simulink model "tbm_ref"  (R2020a)
settings: configuration reference "config_10ms" (kept outside this file)
PreLoadFcn:
  | defParm_cu_tbm_spt
libraries: lib_decmp_Calib_tbm_brkBts_x8 x1, lib_decmp_Calib_tbm_ctr_x8 x1, lib_decmp_CtrSet_tbm_enab_x8 x1, lib_decmp_Calib_tbm_strDistb_x8 x1, lib_decmp_Calib_tbm_supCtr_x8 x1, lib_sig_fault_tolerate x1
settings Model: Creator=Administrator  LastModifiedBy=bowen.zheng
settings ConfigSetRef: SourceName=config_10ms  SourceLocation=Base Workspace

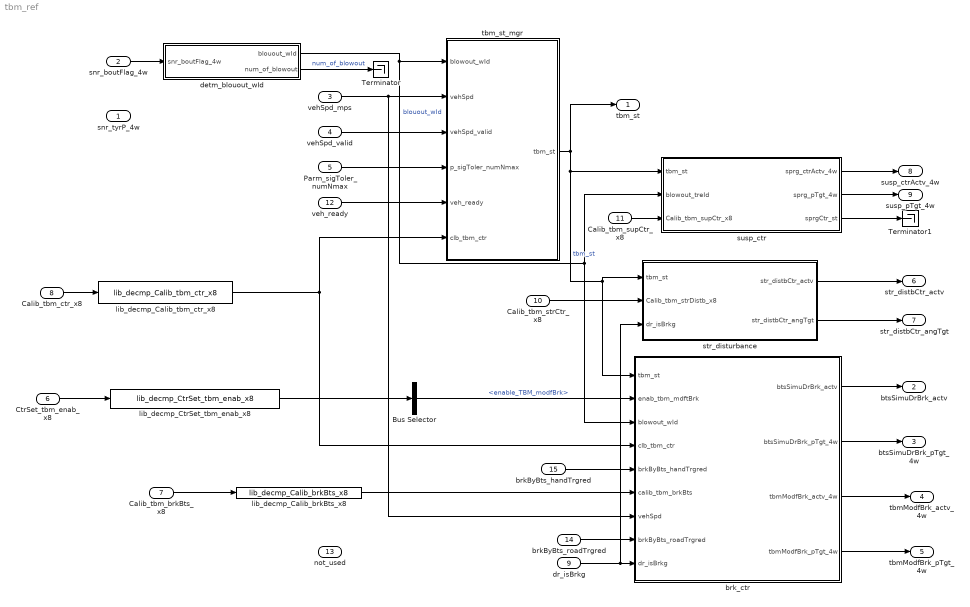
== system tbm_ref ==
  snr_tyrP_4w : Inport  OutDataTypeStr=single  PortDimensions=4
  snr_boutFlag_4w : Inport  Port=2  OutDataTypeStr=boolean  PortDimensions=4
  vehSpd_mps : Inport  Port=3  OutDataTypeStr=single  PortDimensions=1
  vehSpd_valid : Inport  Port=4  OutDataTypeStr=boolean  PortDimensions=1
  Parm_sigToler_numNmax : Inport  Port=5  OutDataTypeStr=int8  PortDimensions=2
  CtrSet_tbm_enab_x8 : Inport  Port=6  OutDataTypeStr=boolean  PortDimensions=8
  Calib_tbm_brkBts_x8 : Inport  Port=7  OutDataTypeStr=single  PortDimensions=8
  Calib_tbm_ctr_x8 : Inport  Port=8  OutDataTypeStr=single  PortDimensions=8
  dr_isBrkg : Inport  Port=9  OutDataTypeStr=boolean
  Calib_tbm_strCtr_x8 : Inport  Port=10  OutDataTypeStr=single  PortDimensions=8
  Calib_tbm_supCtr_x8 : Inport  Port=11  OutDataTypeStr=single  PortDimensions=8
  veh_ready : Inport  Port=12  OutDataTypeStr=boolean
  not_used : Inport  Port=13
  brkByBts_roadTrgred : Inport  Port=14  OutDataTypeStr=boolean
  brkByBts_handTrgred : Inport  Port=15  OutDataTypeStr=boolean  PortDimensions=1
  Bus Selector : BusSelector  OutputSignals=enable_TBM_modfBrk
  Terminator : Terminator
  Terminator1 : Terminator
  brk_ctr : Subsystem
  detm_blouout_wId : MATLAB Function  TreatAsAtomicUnit=on
  lib_decmp_Calib_brkBts_x8 : lib_decmp_Calib_tbm_brkBts_x8/lib_decmp_Calib_brkBts_x8  SystemSampleTime=-1  Latency=0  AutoFrameSizeCalculation=off
  lib_decmp_Calib_tbm_ctr_x8 : lib_decmp_Calib_tbm_ctr_x8/lib_decmp_Calib_tbm_ctr_x8  SystemSampleTime=-1  Latency=0  AutoFrameSizeCalculation=off
  lib_decmp_CtrSet_tbm_enab_x8 : lib_decmp_CtrSet_tbm_enab_x8/lib_decmp_CtrSet_tbm_enab_x8  SystemSampleTime=-1  Latency=0  AutoFrameSizeCalculation=off
  str_disturbance : Subsystem
  susp_ctr : Subsystem
  tbm_st_mgr : Subsystem
  tbm_st : Outport  OutDataTypeStr=Enum: Enum_tbm_tbmSts
  btsSimuDrBrk_actv : Outport  Port=2  OutDataTypeStr=boolean
  btsSimuDrBrk_pTgt_4w : Outport  Port=3  OutDataTypeStr=single  PortDimensions=4
  tbmModfBrk_actv_4w : Outport  Port=4  OutDataTypeStr=boolean  PortDimensions=4
  tbmModfBrk_pTgt_4w : Outport  Port=5  OutDataTypeStr=single  PortDimensions=4
  str_distbCtr_actv : Outport  Port=6  OutDataTypeStr=boolean
  str_distbCtr_angTgt : Outport  Port=7  OutDataTypeStr=single
  susp_ctrActv_4w : Outport  Port=8  OutDataTypeStr=boolean  PortDimensions=4
  susp_pTgt_4w : Outport  Port=9  OutDataTypeStr=single  PortDimensions=4
  wires:
  Calib_tbm_ctr_x8/1 -> lib_decmp_Calib_tbm_ctr_x8/1
  tbm_st_mgr/1(tbm_st) -> tbm_st/1, str_disturbance/1(tbm_st), brk_ctr/1(tbm_st), susp_ctr/1(tbm_st)  "tbm_st"
  snr_boutFlag_4w/1 -> detm_blouout_wId/1(snr_boutFlag_4w)
  vehSpd_mps/1 -> tbm_st_mgr/2(vehSpd), brk_ctr/7(vehSpd)
  vehSpd_valid/1 -> tbm_st_mgr/3(vehSpd_valid)
  Parm_sigToler_numNmax/1 -> tbm_st_mgr/4(p_sigToler_numNmax)
  dr_isBrkg/1 -> str_disturbance/3(dr_isBrkg), brk_ctr/9(dr_isBrkg)
  CtrSet_tbm_enab_x8/1 -> lib_decmp_CtrSet_tbm_enab_x8/1
  lib_decmp_CtrSet_tbm_enab_x8/1 -> Bus Selector/1
  lib_decmp_Calib_tbm_ctr_x8/1 -> tbm_st_mgr/6(clb_tbm_ctr), brk_ctr/4(clb_tbm_ctr)
  detm_blouout_wId/1(blouout_wId) -> brk_ctr/3(blowout_wId), susp_ctr/2(blowout_treId), tbm_st_mgr/1(blowout_wId)  "blouout_wId"
  brkByBts_handTrgred/1 -> brk_ctr/5(brkByBts_handTrgred)
  Calib_tbm_brkBts_x8/1 -> lib_decmp_Calib_brkBts_x8/1
  brk_ctr/1(btsSimuDrBrk_actv) -> btsSimuDrBrk_actv/1
  Calib_tbm_strCtr_x8/1 -> str_disturbance/2(Calib_tbm_strDistb_x8)
  str_disturbance/1(str_distbCtr_actv) -> str_distbCtr_actv/1
  str_disturbance/2(str_distbCtr_angTgt) -> str_distbCtr_angTgt/1
  Calib_tbm_supCtr_x8/1 -> susp_ctr/3(Calib_tbm_supCtr_x8)
  susp_ctr/2(sprg_pTgt_4w) -> susp_pTgt_4w/1
  susp_ctr/1(sprg_ctrActv_4w) -> susp_ctrActv_4w/1
  veh_ready/1 -> tbm_st_mgr/5(veh_ready)
  Bus Selector/1 -> brk_ctr/2(enab_tbm_mdftBrk)  "<enable_TBM_modfBrk>"
  brk_ctr/3(tbmModfBrk_actv_4w) -> tbmModfBrk_actv_4w/1
  brk_ctr/4(tbmModfBrk_pTgt_4w) -> tbmModfBrk_pTgt_4w/1
  brk_ctr/2(btsSimuDrBrk_pTgt_4w) -> btsSimuDrBrk_pTgt_4w/1
  lib_decmp_Calib_brkBts_x8/1 -> brk_ctr/6(calib_tbm_brkBts)
  brkByBts_roadTrgred/1 -> brk_ctr/8(brkByBts_roadTrgred)
  detm_blouout_wId/2(num_of_blowout) -> Terminator/1  "num_of_blowout"
  susp_ctr/3(sprgCtr_st) -> Terminator1/1

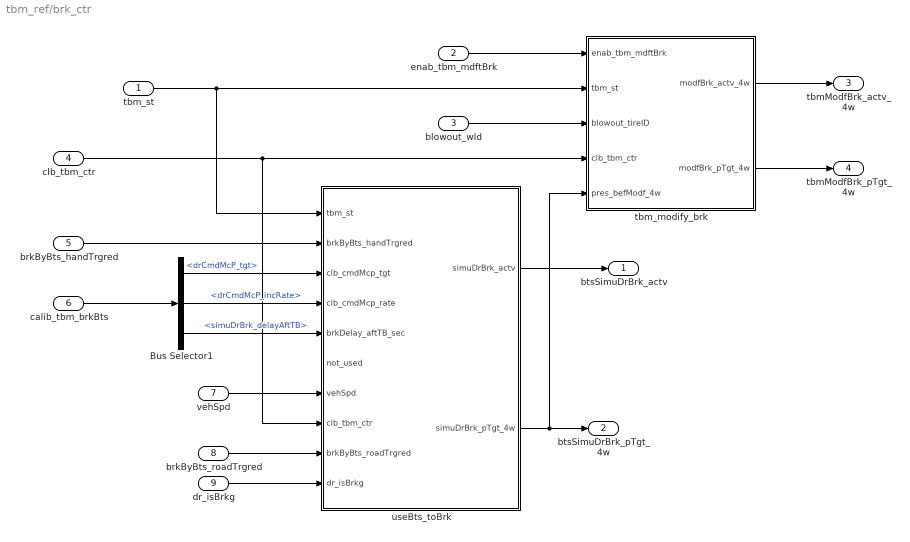
== system tbm_ref/brk_ctr ==
  tbm_st : Inport
  enab_tbm_mdftBrk : Inport  Port=2
  blowout_wId : Inport  Port=3
  clb_tbm_ctr : Inport  Port=4
  brkByBts_handTrgred : Inport  Port=5  OutDataTypeStr=boolean  PortDimensions=1
  calib_tbm_brkBts : Inport  Port=6
  vehSpd : Inport  Port=7  OutDataTypeStr=single  PortDimensions=1
  brkByBts_roadTrgred : Inport  Port=8  OutDataTypeStr=boolean
  dr_isBrkg : Inport  Port=9
  Bus Selector1 : BusSelector  OutputSignals=drCmdMcP_tgt,drCmdMcP_incRate,simuDrBrk_delayAftTB
  tbm_modify_brk : Subsystem
  useBts_toBrk : Subsystem
  btsSimuDrBrk_actv : Outport  OutDataTypeStr=boolean
  btsSimuDrBrk_pTgt_4w : Outport  Port=2  OutDataTypeStr=single  PortDimensions=4
  tbmModfBrk_actv_4w : Outport  Port=3  OutDataTypeStr=boolean  PortDimensions=4
  tbmModfBrk_pTgt_4w : Outport  Port=4  OutDataTypeStr=single  PortDimensions=4
  wires:
  useBts_toBrk/1(simuDrBrk_actv) -> btsSimuDrBrk_actv/1
  clb_tbm_ctr/1 -> useBts_toBrk/8(clb_tbm_ctr), tbm_modify_brk/4(clb_tbm_ctr)
  blowout_wId/1 -> tbm_modify_brk/3(blowout_tireID)
  useBts_toBrk/2(simuDrBrk_pTgt_4w) -> tbm_modify_brk/5(pres_befModf_4w), btsSimuDrBrk_pTgt_4w/1
  Bus Selector1/1 -> useBts_toBrk/3(clb_cmdMcp_tgt)  "<drCmdMcP_tgt>"
  brkByBts_handTrgred/1 -> useBts_toBrk/2(brkByBts_handTrgred)
  calib_tbm_brkBts/1 -> Bus Selector1/1
  tbm_st/1 -> useBts_toBrk/1(tbm_st), tbm_modify_brk/2(tbm_st)
  tbm_modify_brk/2(modfBrk_pTgt_4w) -> tbmModfBrk_pTgt_4w/1
  Bus Selector1/3 -> useBts_toBrk/5(brkDelay_aftTB_sec)  "<simuDrBrk_delayAftTB>"
  Bus Selector1/2 -> useBts_toBrk/4(clb_cmdMcp_rate)  "<drCmdMcP_incRate>"
  enab_tbm_mdftBrk/1 -> tbm_modify_brk/1(enab_tbm_mdftBrk)
  tbm_modify_brk/1(modfBrk_actv_4w) -> tbmModfBrk_actv_4w/1
  vehSpd/1 -> useBts_toBrk/7(vehSpd)
  brkByBts_roadTrgred/1 -> useBts_toBrk/9(brkByBts_roadTrgred)
  dr_isBrkg/1 -> useBts_toBrk/10(dr_isBrkg)

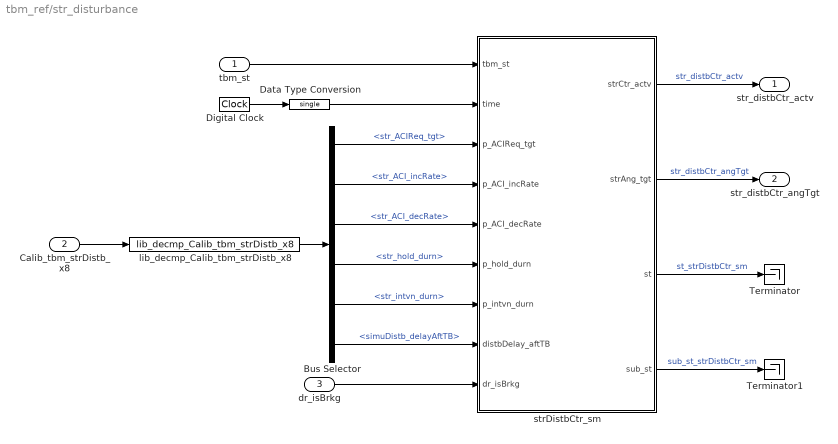
== system tbm_ref/str_disturbance ==
  tbm_st : Inport
  Calib_tbm_strDistb_x8 : Inport  Port=2
  dr_isBrkg : Inport  Port=3
  Bus Selector : BusSelector  OutputSignals=str_ACIReq_tgt,str_ACI_incRate,str_ACI_decRate,str_hold_durn,str_intvn_durn,simuDistb_delayAftTB
  Data Type Conversion : DataTypeConversion  OutDataTypeStr=single
  Digital Clock : DigitalClock  SampleTime=-1
  Terminator : Terminator
  Terminator1 : Terminator
  lib_decmp_Calib_tbm_strDistb_x8 : lib_decmp_Calib_tbm_strDistb_x8/lib_decmp_Calib_tbm_strDistb_x8  SystemSampleTime=-1  Latency=0  AutoFrameSizeCalculation=off
  strDistbCtr_sm : Stateflow chart  TreatAsAtomicUnit=on
  str_distbCtr_actv : Outport  OutDataTypeStr=boolean
  str_distbCtr_angTgt : Outport  Port=2  OutDataTypeStr=single
  wires:
  Digital Clock/1 -> Data Type Conversion/1
  Data Type Conversion/1 -> strDistbCtr_sm/2(time)
  Calib_tbm_strDistb_x8/1 -> lib_decmp_Calib_tbm_strDistb_x8/1
  lib_decmp_Calib_tbm_strDistb_x8/1 -> Bus Selector/1
  Bus Selector/1 -> strDistbCtr_sm/3(p_ACIReq_tgt)  "<str_ACIReq_tgt>"
  Bus Selector/2 -> strDistbCtr_sm/4(p_ACI_incRate)  "<str_ACI_incRate>"
  Bus Selector/3 -> strDistbCtr_sm/5(p_ACI_decRate)  "<str_ACI_decRate>"
  Bus Selector/5 -> strDistbCtr_sm/7(p_intvn_durn)  "<str_intvn_durn>"
  Bus Selector/4 -> strDistbCtr_sm/6(p_hold_durn)  "<str_hold_durn>"
  strDistbCtr_sm/1(strCtr_actv) -> str_distbCtr_actv/1  "str_distbCtr_actv"
  Bus Selector/6 -> strDistbCtr_sm/8(distbDelay_aftTB)  "<simuDistb_delayAftTB>"
  strDistbCtr_sm/2(strAng_tgt) -> str_distbCtr_angTgt/1  "str_distbCtr_angTgt"
  tbm_st/1 -> strDistbCtr_sm/1(tbm_st)
  dr_isBrkg/1 -> strDistbCtr_sm/9(dr_isBrkg)
  strDistbCtr_sm/3(st) -> Terminator/1  "st_strDistbCtr_sm"
  strDistbCtr_sm/4(sub_st) -> Terminator1/1  "sub_st_strDistbCtr_sm"

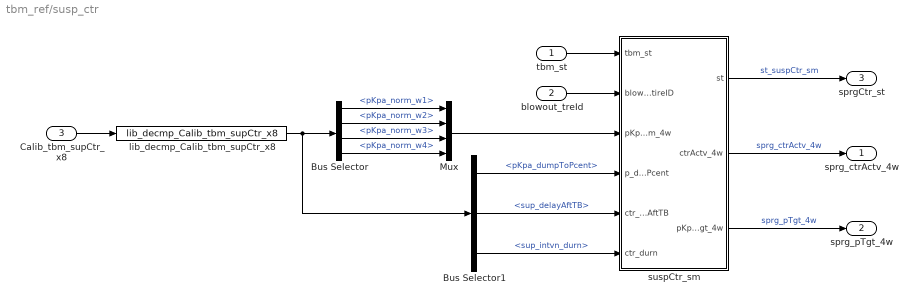
== system tbm_ref/susp_ctr ==
  tbm_st : Inport
  blowout_treId : Inport  Port=2
  Calib_tbm_supCtr_x8 : Inport  Port=3  OutDataTypeStr=single  PortDimensions=8
  Bus Selector : BusSelector  OutputSignals=pKpa_norm_w1,pKpa_norm_w2,pKpa_norm_w3,pKpa_norm_w4
  Bus Selector1 : BusSelector  OutputSignals=pKpa_dumpToPcent,sup_delayAftTB,sup_intvn_durn
  Mux : Mux
  lib_decmp_Calib_tbm_supCtr_x8 : lib_decmp_Calib_tbm_supCtr_x8/lib_decmp_Calib_tbm_supCtr_x8  SystemSampleTime=-1  Latency=0  AutoFrameSizeCalculation=off
  suspCtr_sm : Stateflow chart  TreatAsAtomicUnit=on
  sprg_ctrActv_4w : Outport  OutDataTypeStr=boolean  PortDimensions=4
  sprg_pTgt_4w : Outport  Port=2
  sprgCtr_st : Outport  Port=3
  wires:
  Calib_tbm_supCtr_x8/1 -> lib_decmp_Calib_tbm_supCtr_x8/1
  tbm_st/1 -> suspCtr_sm/1(tbm_st)
  lib_decmp_Calib_tbm_supCtr_x8/1 -> Bus Selector1/1, Bus Selector/1
  Bus Selector/1 -> Mux/1  "<pKpa_norm_w1>"
  Bus Selector/2 -> Mux/2  "<pKpa_norm_w2>"
  Bus Selector/3 -> Mux/3  "<pKpa_norm_w3>"
  Bus Selector/4 -> Mux/4  "<pKpa_norm_w4>"
  Mux/1 -> suspCtr_sm/3(pKpar_nrm_4w)
  blowout_treId/1 -> suspCtr_sm/2(blowout_tireID)
  Bus Selector1/1 -> suspCtr_sm/4(p_dumpToPcent)  "<pKpa_dumpToPcent>"
  Bus Selector1/2 -> suspCtr_sm/5(ctr_delayAftTB)  "<sup_delayAftTB>"
  Bus Selector1/3 -> suspCtr_sm/6(ctr_durn)  "<sup_intvn_durn>"
  suspCtr_sm/2(ctrActv_4w) -> sprg_ctrActv_4w/1  "sprg_ctrActv_4w"
  suspCtr_sm/3(pKpar_tgt_4w) -> sprg_pTgt_4w/1  "sprg_pTgt_4w"
  suspCtr_sm/1(st) -> sprgCtr_st/1  "st_suspCtr_sm"

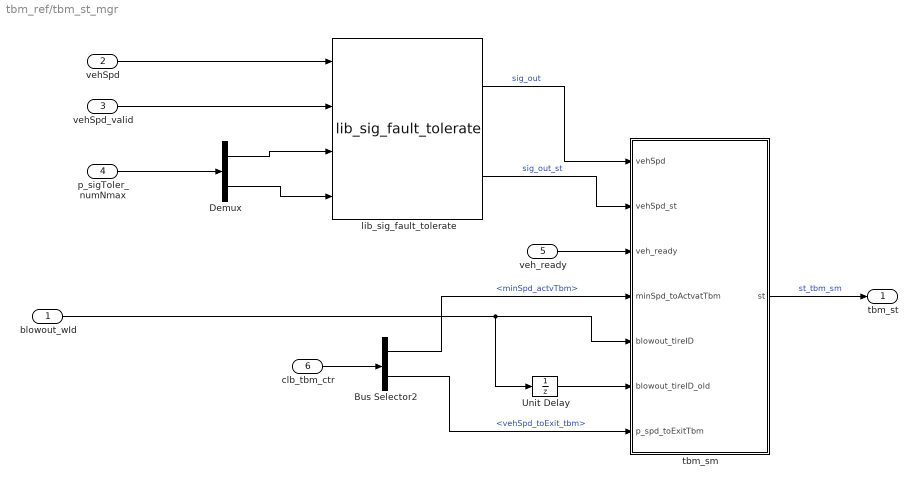
== system tbm_ref/tbm_st_mgr ==
  blowout_wId : Inport
  vehSpd : Inport  Port=2
  vehSpd_valid : Inport  Port=3
  p_sigToler_numNmax : Inport  Port=4
  veh_ready : Inport  Port=5
  clb_tbm_ctr : Inport  Port=6
  Bus Selector2 : BusSelector  OutputSignals=minSpd_actvTbm,vehSpd_toExit_tbm
  Demux : Demux  Outputs=2
  Unit Delay : UnitDelay  SampleTime=-1  HasFrameUpgradeWarning=on
  lib_sig_fault_tolerate : lib_sig_fault_tolerate/lib_sig_fault_tolerate  SystemSampleTime=-1  Latency=0  AutoFrameSizeCalculation=off
  tbm_sm : Stateflow chart  TreatAsAtomicUnit=on
  tbm_st : Outport
  wires:
  blowout_wId/1 -> Unit Delay/1, tbm_sm/5(blowout_tireID)
  lib_sig_fault_tolerate/1 -> tbm_sm/1(vehSpd)  "sig_out"
  veh_ready/1 -> tbm_sm/3(veh_ready)
  lib_sig_fault_tolerate/2 -> tbm_sm/2(vehSpd_st)  "sig_out_st"
  vehSpd_valid/1 -> lib_sig_fault_tolerate/2
  vehSpd/1 -> lib_sig_fault_tolerate/1
  p_sigToler_numNmax/1 -> Demux/1
  Demux/1 -> lib_sig_fault_tolerate/3
  Demux/2 -> lib_sig_fault_tolerate/4
  tbm_sm/1(st) -> tbm_st/1  "st_tbm_sm"
  Unit Delay/1 -> tbm_sm/6(blowout_tireID_old)
  clb_tbm_ctr/1 -> Bus Selector2/1
  Bus Selector2/1 -> tbm_sm/4(minSpd_toActvatTbm)  "<minSpd_actvTbm>"
  Bus Selector2/2 -> tbm_sm/7(p_spd_toExitTbm)  "<vehSpd_toExit_tbm>"

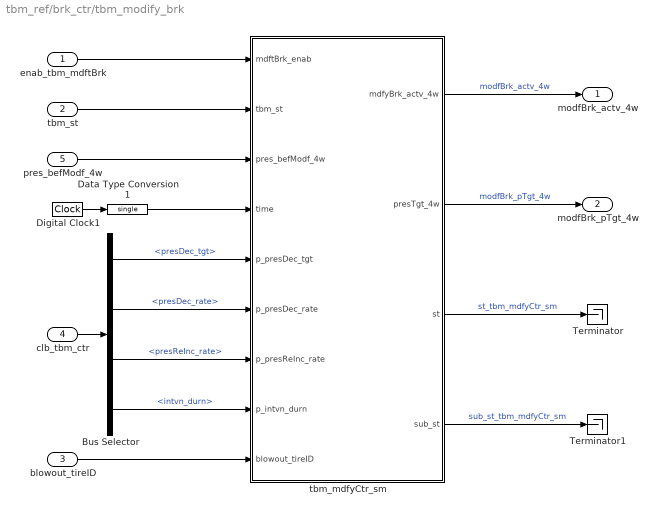
== system tbm_ref/brk_ctr/tbm_modify_brk ==
  enab_tbm_mdftBrk : Inport
  tbm_st : Inport  Port=2
  blowout_tireID : Inport  Port=3
  clb_tbm_ctr : Inport  Port=4  OutDataTypeStr=single  PortDimensions=8
  pres_befModf_4w : Inport  Port=5
  Bus Selector : BusSelector  OutputSignals=presDec_tgt,presDec_rate,presReInc_rate,intvn_durn
  Data Type Conversion1 : DataTypeConversion  OutDataTypeStr=single
  Digital Clock1 : DigitalClock  SampleTime=-1
  Terminator : Terminator
  Terminator1 : Terminator
  tbm_mdfyCtr_sm : Stateflow chart  TreatAsAtomicUnit=on
  modfBrk_actv_4w : Outport  OutDataTypeStr=boolean  PortDimensions=4
  modfBrk_pTgt_4w : Outport  Port=2
  wires:
  tbm_st/1 -> tbm_mdfyCtr_sm/2(tbm_st)
  blowout_tireID/1 -> tbm_mdfyCtr_sm/9(blowout_tireID)
  clb_tbm_ctr/1 -> Bus Selector/1
  Bus Selector/1 -> tbm_mdfyCtr_sm/5(p_presDec_tgt)  "<presDec_tgt>"
  Bus Selector/2 -> tbm_mdfyCtr_sm/6(p_presDec_rate)  "<presDec_rate>"
  Bus Selector/3 -> tbm_mdfyCtr_sm/7(p_presReInc_rate)  "<presReInc_rate>"
  Bus Selector/4 -> tbm_mdfyCtr_sm/8(p_intvn_durn)  "<intvn_durn>"
  Digital Clock1/1 -> Data Type Conversion1/1
  Data Type Conversion1/1 -> tbm_mdfyCtr_sm/4(time)
  pres_befModf_4w/1 -> tbm_mdfyCtr_sm/3(pres_befModf_4w)
  tbm_mdfyCtr_sm/1(mdfyBrk_actv_4w) -> modfBrk_actv_4w/1  "modfBrk_actv_4w"
  tbm_mdfyCtr_sm/2(presTgt_4w) -> modfBrk_pTgt_4w/1  "modfBrk_pTgt_4w"
  enab_tbm_mdftBrk/1 -> tbm_mdfyCtr_sm/1(mdftBrk_enab)
  tbm_mdfyCtr_sm/3(st) -> Terminator/1  "st_tbm_mdfyCtr_sm"
  tbm_mdfyCtr_sm/4(sub_st) -> Terminator1/1  "sub_st_tbm_mdfyCtr_sm"

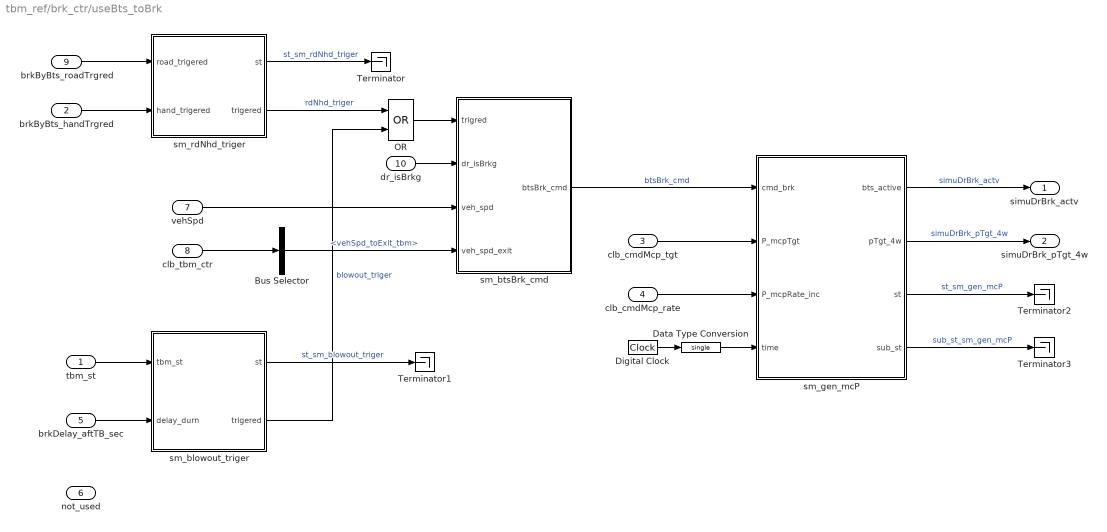
== system tbm_ref/brk_ctr/useBts_toBrk ==
  tbm_st : Inport
  brkByBts_handTrgred : Inport  Port=2
  clb_cmdMcp_tgt : Inport  Port=3
  clb_cmdMcp_rate : Inport  Port=4
  brkDelay_aftTB_sec : Inport  Port=5
  not_used : Inport  Port=6
  vehSpd : Inport  Port=7  OutDataTypeStr=single  PortDimensions=1
  clb_tbm_ctr : Inport  Port=8  OutDataTypeStr=single  PortDimensions=8
  brkByBts_roadTrgred : Inport  Port=9  OutDataTypeStr=boolean
  dr_isBrkg : Inport  Port=10
  Bus Selector : BusSelector  OutputSignals=vehSpd_toExit_tbm
  Data Type Conversion : DataTypeConversion  OutDataTypeStr=single
  Digital Clock : DigitalClock  SampleTime=-1
  OR : Logic  Operator=OR  IconShape=distinctive  AllPortsSameDT=off  OutDataTypeStr=boolean
  Terminator{,1..3} (4 alike) : Terminator
  sm_blowout_triger : Stateflow chart  TreatAsAtomicUnit=on
  sm_btsBrk_cmd : Stateflow chart  TreatAsAtomicUnit=on
  sm_gen_mcP : Stateflow chart  TreatAsAtomicUnit=on
  sm_rdNhd_triger : Stateflow chart  TreatAsAtomicUnit=on
  simuDrBrk_actv : Outport
  simuDrBrk_pTgt_4w : Outport  Port=2
  wires:
  sm_gen_mcP/2(pTgt_4w) -> simuDrBrk_pTgt_4w/1  "simuDrBrk_pTgt_4w"
  brkByBts_handTrgred/1 -> sm_rdNhd_triger/2(hand_trigered)
  Digital Clock/1 -> Data Type Conversion/1
  Data Type Conversion/1 -> sm_gen_mcP/4(time)
  clb_cmdMcp_tgt/1 -> sm_gen_mcP/2(P_mcpTgt)
  sm_gen_mcP/1(bts_active) -> simuDrBrk_actv/1  "simuDrBrk_actv"
  sm_btsBrk_cmd/1(btsBrk_cmd) -> sm_gen_mcP/1(cmd_brk)  "btsBrk_cmd"
  brkDelay_aftTB_sec/1 -> sm_blowout_triger/2(delay_durn)
  sm_blowout_triger/2(trigered) -> OR/2  "blowout_triger"
  clb_cmdMcp_rate/1 -> sm_gen_mcP/3(P_mcpRate_inc)
  tbm_st/1 -> sm_blowout_triger/1(tbm_st)
  vehSpd/1 -> sm_btsBrk_cmd/3(veh_spd)
  clb_tbm_ctr/1 -> Bus Selector/1
  Bus Selector/1 -> sm_btsBrk_cmd/4(veh_spd_exit)  "<vehSpd_toExit_tbm>"
  brkByBts_roadTrgred/1 -> sm_rdNhd_triger/1(road_trigered)
  OR/1 -> sm_btsBrk_cmd/1(trigred)
  sm_rdNhd_triger/2(trigered) -> OR/1  "rdNhd_triger"
  dr_isBrkg/1 -> sm_btsBrk_cmd/2(dr_isBrkg)
  sm_rdNhd_triger/1(st) -> Terminator/1  "st_sm_rdNhd_triger"
  sm_blowout_triger/1(st) -> Terminator1/1  "st_sm_blowout_triger"
  sm_gen_mcP/3(st) -> Terminator2/1  "st_sm_gen_mcP"
  sm_gen_mcP/4(sub_st) -> Terminator3/1  "sub_st_sm_gen_mcP"

== stateflow chart tbm_ref/brk_ctr/tbm_modify_brk/tbm_mdfyCtr_sm ==
  state no_modification
    en:
    st = 0;
    mdfyBrk_actv_4w = [false; false; false; false];
    presTgt_4w = pres_befModf_4w;
    du:
    presTgt_4w = pres_befModf_4w;
  state modification
    en:
    st = 1;
    state pres_dec_and_hold
      en:
      sub_st = 0;
      time_en = time;
      detm_brkMody_4w();
      cal_presTgt_dec_4w();
      du:
      cal_presTgt_dec_4w();
    state pres_reInc
      en:
      sub_st = 2;
      du:
      cal_presTgt_inc_4w();
    pres_dec_and_hold -> pres_reInc : [(time - time_en) > p_intvn_durn ]
  (default) -> no_modification
  no_modification -> pres_dec_and_hold : [       mdftBrk_enab ...
      |   && ( tbm_st == Blowout_mitigate ) ]
  modification -> no_modification : [     ( ~mdftBrk_enab )...
      |    || ( tbm_st ~= Blowout_mitigate ) ]
  data: mdftBrk_enab input boolean; mdfyBrk_actv_4w output boolean size=4; tbm_st input Enum: Enum_tbm_tbmSts; presTgt_4w output single size=4; pres_befModf_4w input single size=4; time input single; p_presDec_tgt input single; p_presDec_rate input single; p_presReInc_rate input single; p_intvn_durn input single; Const_tbmVeh_ctrLoopTime parameter single; time_en local single; st output uint8 size=1; sub_st output uint8 size=1; blowout_tireID input uint8
  function detm_brkMody_4w:
    | function detm_brkMody_4w
    | 
    | mdfyBrk_actv_4w = [false; false; false; false];
    | 
    | if (blowout_tireID == 1 ) || (blowout_tireID == 2 )
    |     mdfyBrk_actv_4w = [true; true; false; false];
    | elseif (blowout_tireID == 3 ) || (blowout_tireID == 4 )  
    |     mdfyBrk_actv_4w = [false; false; true; true];
    | end
  function cal_presTgt_dec_4w:
    | function cal_presTgt_dec_4w
    | 
    | for w = 1:4
    |    if mdfyBrk_actv_4w(w) 
    |        p = presTgt_4w(w) - p_presDec_rate * Const_tbmVeh_ctrLoopTime;       
    |        if  p < min(p_presDec_tgt,  pres_befModf_4w(w))
    |             p = p_presDec_tgt;
    |        end 
    |        presTgt_4w(w) = p;     
    |        
    |        
    |    else
    |        presTgt_4w(w) = pres_befModf_4w(w);
    |    end    
    | end
  function cal_presTgt_inc_4w:
    | function cal_presTgt_inc_4w
    | 
    | for w = 1:4
    |    if mdfyBrk_actv_4w(w) 
    |        p = presTgt_4w(w) + p_presReInc_rate * Const_tbmVeh_ctrLoopTime;
    |        if p > pres_befModf_4w(w)
    |            p = pres_befModf_4w(w);
    |        end     
    |        presTgt_4w(w) = p;
    |        
    |    else
    |        presTgt_4w(w) = pres_befModf_4w(w);
    |    end    
    | end

== stateflow chart tbm_ref/tbm_st_mgr/tbm_sm ==
  state system_init
    en:
    st = Init;
  state watch_for_blowout
    en:
    st = Watch_for_blowout;
  state blowout_mitigation
    en:
    blowout_tireID_en = blowout_tireID;
    st = Blowout_mitigate;
  state terminal
    en:
    st = Blowout_terminal;
  (junction 22) -> system_init : [ vehSpd < p_spd_toExitTbm ]
  (default) -> system_init
  system_init -> (junction 22) [order 1]
  watch_for_blowout -> (junction 22) [order 1]
  system_init -> watch_for_blowout [order 2] : [      veh_ready ...
      |   && ( vehSpd_st == Good )  ...
      |   && ( vehSpd > minSpd_toActvatTbm)  ]
  watch_for_blowout -> system_init [order 2] : [    ~veh_ready ...
      |   ||  ( vehSpd_st == Bad ) ...
      |   || ( vehSpd < 0.95 * minSpd_toActvatTbm ) ]
  watch_for_blowout -> blowout_mitigation [order 3] : [    (    ( blowout_tireID == 1 ) ...
      |        || ( blowout_tireID == 2 ) ...
      |        || ( blowout_tireID == 3 ) ...
      |        || ( blowout_tireID == 4 ) ) ...
      | && ( blowout_tireID_old == 0 ) ]
  blowout_mitigation -> terminal [order 1] : [ vehSpd < p_spd_toExitTbm ]
  blowout_mitigation -> terminal [order 2] : [ blowout_tireID ~= blowout_tireID_en ]
  data: st output Enum: Enum_tbm_tbmSts; vehSpd input single; vehSpd_st input Enum: Enum_sig_status; veh_ready input boolean; minSpd_toActvatTbm input single; blowout_tireID input uint8; blowout_tireID_old input uint8; blowout_tireID_en local uint8; p_spd_toExitTbm input single

== stateflow chart tbm_ref/susp_ctr/suspCtr_sm ==
  state no_ctr
    en:
    st = 0;
    ctrActv_4w = [false; false; false; false];
    pKpar_tgt_4w = pKpar_nrm_4w;
  state delay
    en:
    st = 1;
  state ctr
    en:
    st = 2;
    detm_actvNtgt_4w();
  state end_ctr
    en:
    st = 3;
    ctrActv_4w = [false; false; false; false];
  (default) -> no_ctr
  (junction 21) -> no_ctr : [ Blowout_mitigate ~= tbm_st]
  delay -> (junction 21) [order 1]
  ctr -> (junction 21) [order 2]
  no_ctr -> delay : [ Blowout_mitigate == tbm_st]
  delay -> ctr [order 2] : after (ctr_delayAftTB, sec)
  ctr -> end_ctr [order 1] : after (ctr_durn, sec)
  data: st output uint8; tbm_st input Enum: Enum_tbm_tbmSts; blowout_tireID input uint8; ctrActv_4w output boolean size=4; pKpar_nrm_4w input single; pKpar_tgt_4w output single; p_dumpToPcent input single; ctr_delayAftTB input single; ctr_durn input single
  function detm_actvNtgt_4w:
    | function detm_actvNtgt_4w
    | 
    | % ctrActv_4w = [false; false; false; false];
    | % pKpar_tgt_4w = pKpar_nrm_4w;
    | 
    |     if (1 == blowout_tireID) || (4 == blowout_tireID )
    |       set_pTgt(2);
    |       set_pTgt(3);
    | 
    |     elseif (blowout_tireID == 2 ) || (blowout_tireID == 3 ) 
    |       set_pTgt(1);
    |       set_pTgt(4);
    | 
    |     end
    | 
    | 
    | end
    | 
    | 
    | % if (1 == blowout_tireID) || (4 == blowout_tireID )
    | %    w = 2;
    | %    ctrActv_4w(w) = true; 
    | %    pKpar_tgt_4w(w) = pKpar_nrm_4w(w) * p_dumpToPcent;
    | %    
    | %    w = 3;
    | %    ctrActv_4w(w) = true; 
    | %    pKpar_tgt_4w(w) = pKpar_nrm_4w(w) * p_dumpToPcent;
    | %    
    | % elseif (blowout_tireID == 2 ) || (blowout_tireID == 3 ) 
    | %     w = 1;
    | %    ctrActv_4w(w) = true; 
    | %    pKpar_tgt_4w(w) = pKpar_nrm_4w(w) * p_dumpToPcent;
    | %    
    | %    w = 4;
    | %    ctrActv_4w(w) = true; 
    | %    pKpar_tgt_4w(w) = pKpar_nrm_4w(w) * p_dumpToPcent;
    | %    
    | % end
    | 
    | function set_pTgt( w )
    |    ctrActv_4w(w) = true; 
    |    pKpar_tgt_4w(w) = pKpar_nrm_4w(w) * p_dumpToPcent;
    | end

== matlab function tbm_ref/detm_blouout_wId ==
  data: snr_boutFlag_4w input boolean size=4; blouout_wId output uint8 size=1; num_of_blowout output uint8 size=1
function [blouout_wId,num_of_blowout] = fcn(snr_boutFlag_4w)


blouout_wId = uint8(0);
num_of_blowout = uint8(0);

for w = uint8(1) : 4
    if snr_boutFlag_4w (w) 
        blouout_wId = w;
        num_of_blowout = num_of_blowout + 1;
    end
    
end

if num_of_blowout ~= 1   % overwrite blowout_wId
    blouout_wId = uint8(0);    
end

== stateflow chart tbm_ref/brk_ctr/useBts_toBrk/sm_gen_mcP ==
  state no_simuDrBrk
    en:
    st = 0;
    bts_active = false;
    pTgt_4w = [0; 0; 0; 0];
  state simuDrBrk
    en:
    st = 1;
    bts_active = true;
    state inc_mcP
      en:
      sub_st = 0;
      time_en = time;
      mcpTgt = ( time - time_en ) * P_mcpRate_inc;
      pTgt_4w = [mcpTgt; mcpTgt; mcpTgt; mcpTgt];
      du:
      mcpTgt = ( time - time_en ) * P_mcpRate_inc;
      pTgt_4w = [mcpTgt; mcpTgt; mcpTgt; mcpTgt];
    state hold_mcP
      en:
      sub_st = 1;
      mcpTgt = P_mcpTgt;
      pTgt_4w = [mcpTgt; mcpTgt; mcpTgt; mcpTgt];
    (default) -> inc_mcP
    inc_mcP -> hold_mcP : [ mcpTgt >= P_mcpTgt ]
  (default) -> no_simuDrBrk
  no_simuDrBrk -> simuDrBrk : [ cmd_brk ]
  simuDrBrk -> no_simuDrBrk : [ ~cmd_brk]
  data: cmd_brk input boolean; bts_active output boolean; P_mcpTgt input single; P_mcpRate_inc input single; time input single; time_en local single; pTgt_4w output single size=4; st output uint8; sub_st output uint8 size=1; mcpTgt local single

== stateflow chart tbm_ref/brk_ctr/useBts_toBrk/sm_blowout_triger ==
  state no_brk
    en:
    st = 0;
    trigered = false;
  state pending_brk
    en:
    st = 1;
    trigered = false;
  state brk
    en:
    st = 2;
    trigered = true;
  (default) -> no_brk
  (junction 16) -> no_brk : [ Blowout_mitigate ~= tbm_st ]
  no_brk -> pending_brk : [ Blowout_mitigate == tbm_st]
  pending_brk -> (junction 16) [order 1]
  brk -> (junction 16)
  pending_brk -> brk [order 2] : after(delay_durn, sec)
  data: tbm_st input Enum: Enum_tbm_tbmSts; delay_durn input single; st output uint8; trigered output boolean

== stateflow chart tbm_ref/brk_ctr/useBts_toBrk/sm_rdNhd_triger ==
  state waiting
    en:
    st = 0;
    trigered = false;
  state triggered
    en:
    st = 1;
    trigered = true;
  (default) -> waiting
  waiting -> triggered : [ road_trigered ||  hand_trigered ]
  triggered -> waiting : [       ( ~road_trigered )...
      |   && ( ~hand_trigered ) ]
  data: st output uint8; road_trigered input boolean; hand_trigered input boolean; trigered output boolean

== stateflow chart tbm_ref/brk_ctr/useBts_toBrk/sm_btsBrk_cmd ==
  state no_brk
    en:
    btsBrk_cmd = false;
  state brk
    en:
    btsBrk_cmd = true;
  (default) -> no_brk
  no_brk -> brk : [ trigred ...
      |  && ( ~dr_isBrkg) ]
  brk -> no_brk : [ dr_isBrkg || ( veh_spd < veh_spd_exit ) ]
  data: btsBrk_cmd output boolean; trigred input boolean; dr_isBrkg input boolean; veh_spd input single; veh_spd_exit input single

== stateflow chart tbm_ref/str_disturbance/strDistbCtr_sm ==
  state gen_disturbance
    en:
    st = 2;    time_enDistb = time;
    strCtr_actv = true;
    state Ramp_hold
      en:
      sub_st = 1; time_enDistbHold = time;
      strAng_tgt = p_ACIReq_tgt;
      du:
      strAng_tgt = p_ACIReq_tgt;
    state Ramp_inc
      en:
      sub_st = 0;
      strAng_tgt = strAng_tgt + p_ACI_incRate * Const_tbmVeh_ctrLoopTime;
      strAng_tgt = min( p_ACIReq_tgt, strAng_tgt );
      du:
      strAng_tgt = strAng_tgt + p_ACI_incRate * Const_tbmVeh_ctrLoopTime;
      strAng_tgt = min( p_ACIReq_tgt, strAng_tgt );
    state Ramp_dec
      en:
      sub_st = 2;
      du:
      strAng_tgt = strAng_tgt - p_ACI_decRate * Const_tbmVeh_ctrLoopTime;
      strAng_tgt = max( 0, strAng_tgt );
    Ramp_inc -> Ramp_hold : [strAng_tgt >= p_ACIReq_tgt]
    Ramp_hold -> Ramp_dec : [(time - time_enDistbHold) > p_hold_durn]
  state init
    en:
    st = 0;
    strCtr_actv = false;
    strAng_tgt = 0;
  state delay
    en:
    st = 1;
    strCtr_actv = false;
    strAng_tgt = 0;
  state end
    en:
    st = 3;
    strCtr_actv = false;
    strAng_tgt = 0;
  (default) -> init
  init -> delay : [ Blowout_mitigate == tbm_st]
  (junction 58) -> init : [ Blowout_mitigate ~= tbm_st ]
  gen_disturbance -> (junction 58) [order 2]
  delay -> (junction 58) [order 1]
  delay -> Ramp_inc [order 2] : after(distbDelay_aftTB, sec)
  gen_disturbance -> end [order 1] : [  dr_isBrkg ...
      |    || ( (time - time_enDistb) > p_intvn_durn ) ]
  data: tbm_st input Enum: Enum_tbm_tbmSts; strCtr_actv output boolean; time input single; strAng_tgt output single; Const_tbmVeh_ctrLoopTime parameter single; p_ACIReq_tgt input single; p_ACI_incRate input single; p_ACI_decRate input single; p_hold_durn input single; p_intvn_durn input single; time_enDistb local single; st output uint8 size=1; sub_st output uint8 size=1; time_enDistbHold local single; distbDelay_aftTB input single; dr_isBrkg input boolean
